simulink library "see_saw"  (R2013b)
settings: Solver=ode45  StartTime=0.0  StopTime=10.0  RelTol=1e-3
undefined symbols (not defined in the file): DiscIntNeverNeededParam, gcbh, K, R, realtime
libraries: legonxtlib x9
(part 2 of 2)

== stateflow chart see_saw/see_saw_mode_o ==
  state see_saw_mode
    entry:
    desired_tail = single(1.6);
    during:
    normalizedLight = processLight(sensors.light,lightCalib);
    PWM.tail = tail_controller(sensors.theta_T, desired_tail);
    DispTheta(states.phi);
    state light = processLight(rawLight,lightCalib) [function]
    state StandUp
      entry: debugFlag = uint16(602);
      initFlags.theta = single(1);
      initFlags.gyroReset = single(1);
      during:
      desired_tail = desired_tail + single(0.0008);
    state DispTheta(theta) [function]
    state cmd = phiController(phi,desiredPhi,battery) [function]
    state Balancing
      state SeesawLogic [parallel]
        settings: executionOrder=2
        state StationnaryBalance
          entry: debugFlag = uint16(603);
          desired_tail = single(0.5);
          initFlags.theta = single(0);
          initFlags.gyroReset = single(0);
          desired_states = balancerStates_Bus0;
        state Approach
          entry: debugFlag = uint16(604);
          during:
          turningPWM = lineTracker(single(-0.3), normalizedLight, single(1.3), sensors.battery);
          exit:
          turningPWM = single(0);
          state StartWalking
            entry:
            entry: debugFlag = uint16(605);
            des_vel = single(0.04);
            during:
            des_vel = des_vel+single(0.00024);
          state Walk
            entry: debugFlag = uint16(605);
          (default) -> StartWalking
          StartWalking -> Walk : [des_vel >= single(0.1)]
        state Seesaw
          state JumpOnIt
            entry:
            Speak;
            debugFlag = uint16(606);
            theta_ref = states.balancerStates.theta;
            phi_ref = states.phi;
            des_vel = single(0.15);
          state OnSeeSaw
            during:
            turningPWM = phiController(states.phi, phi_ref, sensors.battery);
            state GoingUP
              entry:
              entry: debugFlag = uint16(607);
              des_vel = single(0.1);
            state GoingBack
              entry:
              entry: debugFlag = uint16(608);
              des_vel = single(-0.1);
            state GoUpAgain
              entry:
              entry: debugFlag = uint16(609);
              des_vel = single(0.05);
              during:
              des_vel = des_vel + single(0.00024);
            state WaitForGettingDown
            GoingUP -> GoingBack : [states.balancerStates.theta >= theta_ref + single(9)]
            GoingBack -> GoUpAgain : [states.balancerStates.theta <= theta_ref + single(8.2)]
            GoUpAgain -> WaitForGettingDown : [des_vel >= 0.075]
          state Stop
            entry: debugFlag = uint16(610);
            des_vel = single(0.1);
            during:
            turningPWM = lineTracker(single(-0.3), normalizedLight, single(1.3), sensors.battery);
          state Warning
            entry: debugFlag = uint16(621);
            des_vel = single(0.1);
            during:
            turningPWM = lineTracker(single(-0.3), normalizedLight, single(1.3), sensors.battery);
          state DoneStates
            du: turningPWM = lineTracker(single(-0.3), normalizedLight, single(1.3), sensors.battery);
            state Done
              entry: debugFlag = uint16(611);
            state DecreaseSpeed
              en: des_vel = single(0.05);
              entry: debugFlag = uint16(612);
              du:
              des_vel = des_vel -single(0.0004);
            state ExitSeeSaw
              en:
              des_vel = single(0.025);
            Done -> DecreaseSpeed : [after(2,sec)]
            DecreaseSpeed -> ExitSeeSaw : [des_vel<single(0.025)]
          state Woops
            state Stabilize
              en:debugFlag = uint16(1120);
            state BackUpB1
              en: des_vel = single(-0.04);
              en:debugFlag = uint16(1121);
            state ReachedLine
              en:
              theta_l_0 = sensors.theta_L;
              debugFlag = uint16(1122);
              phi_ref = states.phi;
            state TurnNow
              en:
              des_vel = single(0);
              debugFlag = uint16(1123);
              des_turning = single(1.65);
              du:
              turningPWM = phiController(states.phi, (phi_ref - des_turning), sensors.battery);
            state GoOnYourMerryWay
              en:
              des_vel = single(0.02);
              %tracking = uint8(1);
              du:
              des_vel = des_vel+single(0.0004);
              turningPWM = lineTracker(single(-0.3), normalizedLight, single(1.3), sensors.battery);
              debugFlag = uint16(1124);
            (default) -> Stabilize : {FoundLine =uint8( 0);
                | %tracking = uint8(0);
                | %des_turning = single(0);
                | turningPWM = single(0);
                | des_vel = single(0);
                | }
            BackUpB1 -> ReachedLine : [normalizedLight >= single(0.5) ]
            Stabilize -> BackUpB1 : after(2,sec)
            ReachedLine -> TurnNow : [sensors.theta_L < theta_l_0-single(0.5)]
            TurnNow -> GoOnYourMerryWay : after(2.5,sec)
          (default) -> JumpOnIt
          JumpOnIt -> GoingUP : [states.balancerStates.theta >= theta_ref+single(1.57)]
          GoOnYourMerryWay -> ExitSeeSaw : [des_vel >=  single(0.025)]
          WaitForGettingDown -> Stop : [states.balancerStates.theta >= theta_ref + single(17)]
          Stop -> Warning [order 1] : [states.phi - phi_ref > single(0.5)]
          Warning -> Done [order 1] : [states.phi - phi_ref < single(-0.5)]
          Stop -> Done [order 2] : [states.phi - phi_ref < single(-0.5)]
          Warning -> Woops [order 2] : [states.phi - phi_ref > single(1.7)]
        state RaceDone
          entry: debugFlag = uint16(599);
          current_mode_status = OperationModeStatusEnum.SUCCESSFULLY_COMPLETED;
        (default) -> StationnaryBalance
        StationnaryBalance -> Approach : after(2,sec)
        Approach -> Seesaw : [states.balancerStates.theta_dot<single(-4)  && states.theta_dot_dot < single(-60) ]
        ExitSeeSaw -> RaceDone : after(0.5, sec)
      state After [parallel]
        during:
        forwardPWM = balance_ctrl(states.balancerStates, des_vel ,sensors.battery)
        PWM.left = forwardPWM - turningPWM;
        PWM.right = forwardPWM + turningPWM;
        settings: executionOrder=1
    state cmd = lineTracker(desiredLight,light,trackingPower,battery) [function]
    state Speak [function]
    state cmd = tail_controller(current,desired) [function]
    state cmd = balance_ctrl(balancerStates,desired_velocity,battery) [function]
    (default) -> StandUp
    StandUp -> Balancing : [desired_tail >=single(2.0) && sensors.theta_T >= single(2.0)]
  data: rawLight function_input single size=1; lightCalib function_input Bus: Light_Bus size=1; light function_output; theta function_input double size=1; cmd function_output; phi function_input single size=1; desiredPhi function_input single size=1; battery function_input double size=1; cmd function_output single size=1; desiredLight function_input single size=1; light function_input single size=1; trackingPower function_input single size=1; battery function_input double size=1; current function_input single size=1; desired function_input single size=1; cmd function_output single size=1; balancerStates function_input Bus: Balancer_States_Bus size=1; desired_velocity function_input single size=1; battery function_input double size=1; cmd function_output single size=1; states input Bus: States_Bus size=1; sensors input Bus: Sensors_Bus size=1; PWM output Bus: PWM_bus size=1; initFlags output Bus: Init_Bus size=1; debugFlag output uint16 size=1; desired_states local Bus: Balancer_States_Bus size=1; desired_tail local single size=1; current_mode_status data_store_memory; balancerStates_Bus0 parameter Bus: Balancer_States_Bus size=1; lightCalib data_store_memory; normalizedLight local single size=1; des_vel local single size=1; theta_ref local single size=1; forwardPWM local single size=1; turningPWM local single size=1; phi_ref local single; FoundLine local; des_turning local; theta_l_0 local

== stateflow chart see_saw/see_saw ==
  state see_saw_mode
    entry:
    desired_tail = single(1.6);
    desired_psi = single(0);
    theta_ref = single(0);
    during:
    normalizedLight = processLight(sensors.light,lightCalib);
    PWM.tail = tail_controller(sensors.theta_T, desired_tail);
    DispTheta(normalizedLight,turningPWM);
    state light = processLight(rawLight,lightCalib) [function]
    state StandUp
      entry: debugFlag = uint16(602);
      initFlags.theta = single(1);
      initFlags.gyroReset = single(1);
      during:
      desired_tail = desired_tail + single(0.0008);
    state DispTheta(light,turningPWM) [function]
    state cmd = phiController(phi,desiredPhi,battery) [function]
    state Balancing
      state SeesawLogic [parallel]
        settings: executionOrder=2
        state StationnaryBalance
          entry: debugFlag = uint16(603);
          desired_tail = single(0.5);
          initFlags.theta = single(0);
          initFlags.gyroReset = single(0);
          desired_states = balancerStates_Bus0;
        state Approach
          entry: debugFlag = uint16(604);
          during:
          turningPWM = lineTracker(single(-0.3), normalizedLight, single(1.3), sensors.battery);
          exit:
          turningPWM = single(0);
          state StartWalking
            entry:
            entry: debugFlag = uint16(605);
            des_vel = single(0.04);
            during:
            des_vel = des_vel+single(0.00024);
          state Walk
            entry: debugFlag = uint16(605);
          (default) -> StartWalking
          StartWalking -> Walk : [des_vel >= single(0.1)]
        state Seesaw
          state JumpOnIt
            entry:
            Speak;
            debugFlag = uint16(606);
            theta_ref = states.balancerStates.theta;
            phi_ref = states.phi;
            des_vel = single(0.15);
          state OnSeeSaw
            state GoingUP
              entry:
              debugFlag = uint16(607);des_vel = single(0.07);
              during:
              turningPWM = lineTracker(single(-0.6), normalizedLight, single(1), sensors.battery) + ...
              phiController(states.phi, phi_ref, sensors.battery);
            state GoingBack
              entry:
              debugFlag = uint16(608);
              des_vel = single(-0.1);
              during:
              turningPWM =phiController(states.phi, phi_ref, sensors.battery);
            state GoUpAgain
              entry:
              entry: debugFlag = uint16(609);
              des_vel = single(0.07);
              during:
              turningPWM = lineTracker(single(-0.6), normalizedLight, single(1), sensors.battery) + ...
              phiController(states.phi, phi_ref, sensors.battery);
              %des_vel = des_vel + single(0.00024);
            state WaitForGettingDown
              during:
              turningPWM = lineTracker(single(-0.6), normalizedLight, single(1), sensors.battery) + ...
              phiController(states.phi, phi_ref, sensors.battery);
            GoingUP -> GoingBack : [states.balancerStates.theta >= theta_ref + single(9.2)]
            GoingBack -> GoUpAgain : [states.balancerStates.theta <= theta_ref + single(8.2)]
          state Stop
            entry: debugFlag = uint16(610);
            des_vel = single(0.1);
            during:
            turningPWM = lineTracker(single(-0.3), normalizedLight, single(1.3), sensors.battery)+ ...
            phiController(states.phi, phi_ref, sensors.battery);
          state Warning
            entry: debugFlag = uint16(621);
            des_vel = single(0.05);
            during:
            turningPWM = lineTracker(single(-0.3), normalizedLight, single(1.6), sensors.battery);
          state DoneStates
            du: turningPWM = lineTracker(single(-0.3), normalizedLight, single(1.3), sensors.battery)+ ...
            phiController(states.phi, phi_ref, sensors.battery);
            state Done
              entry: debugFlag = uint16(611);
            state DecreaseSpeed
              en: des_vel = single(0.08);
              entry: debugFlag = uint16(612);
              du:
              des_vel = des_vel -single(0.0004);
            state ExitSeeSaw
              en:
              des_vel = single(0.08)
            Done -> DecreaseSpeed : [after(2,sec)]
            DecreaseSpeed -> ExitSeeSaw : %[des_vel<single(0.08)]
          state Woops
            state Stabilize
              en:debugFlag = uint16(1120);
            state BackUpB1
              en: des_vel = single(-0.05);
              en:debugFlag = uint16(1121);
            state ReachedLine
              en:
              theta_l_0 = sensors.theta_L;
              debugFlag = uint16(1122);
              phi_ref = states.phi;
            state TurnNow
              en:
              des_vel = single(0);
              debugFlag = uint16(1123);
              des_turning = single(1.65);
              du:
              turningPWM = phiController(states.phi, (phi_ref - des_turning), sensors.battery);
            state GoOnYourMerryWay
              en:
              des_vel = single(0.02);
              turningPWM = lineTracker(single(-0.3), normalizedLight, single(1.3), sensors.battery);
              du:
              des_vel = des_vel+single(0.0004);
              turningPWM = lineTracker(single(-0.3), normalizedLight, single(1.3), sensors.battery);
              debugFlag = uint16(1124);
            (default) -> Stabilize : {FoundLine =uint8( 0);
                | %tracking = uint8(0);
                | %des_turning = single(0);
                | turningPWM = single(0);
                | des_vel = single(0);
                | }
            BackUpB1 -> ReachedLine : [normalizedLight >= single(0.5) ]
            Stabilize -> BackUpB1 : after(2,sec)
            ReachedLine -> TurnNow : [sensors.theta_L < theta_l_0-single(0.5)]
            TurnNow -> GoOnYourMerryWay : after(2.5,sec)
          (default) -> JumpOnIt
          JumpOnIt -> GoingUP : [states.balancerStates.theta >= theta_ref+single(1.57)]
          GoUpAgain -> Stop : [states.balancerStates.theta >= theta_ref + single(17)]
          GoOnYourMerryWay -> ExitSeeSaw : [des_vel >=  single(0.04)]
          Stop -> Warning [order 1] : [states.phi - phi_ref > single(0.5)]
          Warning -> Done [order 1] : [states.phi - phi_ref < single(-0.2)]
          Stop -> Done [order 2] : [states.phi - phi_ref < single(0)]
          Warning -> Woops [order 2] : [states.phi - phi_ref > single(1.7)]
        state Parking
          en,du:
          turningPWM = single(2)*lineTracker(single(-0.3), normalizedLight, single(1), sensors.battery) + phiController(states.phi, phi_ref, sensors.battery);
          state DropTailAndGrey
            state TailDrop
              entry: debugFlag = uint16(801);
              during:
              desired_tail = desired_tail + single(0.1);
            state LookForGrey
              entry: debugFlag = uint16(803);
            (default) -> TailDrop
            TailDrop -> LookForGrey : [desired_tail > single(1.6)]
          state WaitAndCount
            entry: debugFlag = uint16(804);
          state FallBack
            entry: debugFlag = uint16(805);
            desired_psi = single(-0.15);
          state DoneWithParking
            entry: debugFlag = uint16(806);
            exit:
            PWM.left = single(0);
            PWM.right = single(0);
          (default) -> DropTailAndGrey
          LookForGrey -> FallBack : [states.balancerStates.theta >= theta_ref + single(32)]
          WaitAndCount -> WaitAndCount [order 1] : [-100*normalizedLight <= single(-12)]
          WaitAndCount -> FallBack [order 2] : after(0.3,sec)
          FallBack -> DoneWithParking : after(0.2,sec)
        state RaceDone
          entry: debugFlag = uint16(599);
          current_mode_status = OperationModeStatusEnum.SUCCESSFULLY_COMPLETED;
        (default) -> StationnaryBalance
        StationnaryBalance -> Approach : after(2,sec)
        Approach -> Seesaw : [states.balancerStates.theta_dot<single(-4)  && states.theta_dot_dot < single(-60) ]
        ExitSeeSaw -> Parking : after(0.1,sec)
      state After [parallel]
        during:
        forwardPWM = balance_ctrl(states.balancerStates, des_vel ,sensors.battery, desired_psi)
        if (debugFlag~= uint16(806))
        PWM.left = forwardPWM - turningPWM;
        PWM.right = forwardPWM + turningPWM;
        else
        PWM.left = single(0);
        PWM.right = single(0);
        end
        settings: executionOrder=1
    state cmd = lineTracker(desiredLight,light,trackingPower,battery) [function]
    state Speak [function]
    state cmd = tail_controller(current,desired) [function]
    state cmd = balance_ctrl(balancerStates,desired_velocity,battery,desired_psi) [function]
    (default) -> StandUp
    StandUp -> Balancing : [desired_tail >=single(2.0) && sensors.theta_T >= single(2.0)]
  data: rawLight function_input single size=1; lightCalib function_input Bus: Light_Bus size=1; light function_output; light function_input double size=1; turningPWM function_input double size=1; cmd function_output; phi function_input single size=1; desiredPhi function_input single size=1; battery function_input double size=1; cmd function_output single size=1; desiredLight function_input single size=1; light function_input single size=1; trackingPower function_input single size=1; battery function_input double size=1; current function_input single size=1; desired function_input single size=1; cmd function_output single size=1; balancerStates function_input Bus: Balancer_States_Bus size=1; desired_velocity function_input single size=1; battery function_input double size=1; cmd function_output single size=1; desired_psi function_input single size=1; states input Bus: States_Bus size=1; sensors input Bus: Sensors_Bus size=1; PWM output Bus: PWM_bus size=1; initFlags output Bus: Init_Bus size=1; debugFlag output uint16 size=1; desired_states local Bus: Balancer_States_Bus size=1; desired_tail local single size=1; current_mode_status data_store_memory; balancerStates_Bus0 parameter Bus: Balancer_States_Bus size=1; lightCalib data_store_memory; normalizedLight local single size=1; des_vel local single size=1; theta_ref local single size=1; forwardPWM local single size=1; turningPWM local single size=1; phi_ref local single; FoundLine local; des_turning local; theta_l_0 local; desired_psi local

== stateflow chart see_saw/see_saw_8262013 ==
  state see_saw_mode
    entry:
    desired_tail = single(1.6);
    desired_psi = single(0);
    theta_ref = single(0);
    during:
    normalizedLight = processLight(sensors.light,lightCalib);
    PWM.tail = tail_controller(sensors.theta_T, desired_tail);
    DispTheta(states.balancerStates.theta - theta_ref);
    state light = processLight(rawLight,lightCalib) [function]
    state StandUp
      entry: debugFlag = uint16(602);
      initFlags.theta = single(1);
      initFlags.gyroReset = single(1);
      during:
      desired_tail = desired_tail + single(0.0008);
    state DispTheta(theta) [function]
    state cmd = phiController(phi,desiredPhi,battery) [function]
    state Balancing
      state SeesawLogic [parallel]
        settings: executionOrder=2
        state StationnaryBalance
          entry: debugFlag = uint16(603);
          desired_tail = single(0.5);
          initFlags.theta = single(0);
          initFlags.gyroReset = single(0);
          desired_states = balancerStates_Bus0;
        state Approach
          entry: debugFlag = uint16(604);
          during:
          turningPWM = lineTracker(single(-0.3), normalizedLight, single(1.3), sensors.battery);
          exit:
          turningPWM = single(0);
          state StartWalking
            entry:
            entry: debugFlag = uint16(605);
            des_vel = single(0.04);
            during:
            des_vel = des_vel+single(0.00024);
          state Walk
            entry: debugFlag = uint16(605);
          (default) -> StartWalking
          StartWalking -> Walk : [des_vel >= single(0.1)]
        state Seesaw
          state JumpOnIt
            entry:
            Speak;
            debugFlag = uint16(606);
            theta_ref = states.balancerStates.theta;
            phi_ref = states.phi;
            des_vel = single(0.15);
          state OnSeeSaw
            during:
            turningPWM = phiController(states.phi, phi_ref, sensors.battery);
            state GoingUP
              entry:
              entry: debugFlag = uint16(607);
              des_vel = single(0.1);
            state GoingBack
              entry:
              entry: debugFlag = uint16(608);
              des_vel = single(-0.1);
            state GoUpAgain
              entry:
              entry: debugFlag = uint16(609);
              des_vel = single(0.05);
              during:
              des_vel = des_vel + single(0.00024);
            state WaitForGettingDown
            GoingUP -> GoingBack : [states.balancerStates.theta >= theta_ref + single(9)]
            GoingBack -> GoUpAgain : [states.balancerStates.theta <= theta_ref + single(8.2)]
            GoUpAgain -> WaitForGettingDown : [des_vel >= 0.075]
          state Stop
            entry: debugFlag = uint16(610);
            des_vel = single(0.1);
            during:
            turningPWM = lineTracker(single(-0.3), normalizedLight, single(1.3), sensors.battery);
          state Warning
            entry: debugFlag = uint16(621);
            des_vel = single(0.05);
            during:
            turningPWM = lineTracker(single(-0.3), normalizedLight, single(1.6), sensors.battery);
          state DoneStates
            du: turningPWM = lineTracker(single(-0.3), normalizedLight, single(1.3), sensors.battery);
            state Done
              entry: debugFlag = uint16(611);
            state DecreaseSpeed
              en: des_vel = single(0.08);
              entry: debugFlag = uint16(612);
              du:
              des_vel = des_vel -single(0.0004);
            state ExitSeeSaw
              en:
              des_vel = single(0.08)
            Done -> DecreaseSpeed : [after(2,sec)]
            DecreaseSpeed -> ExitSeeSaw : %[des_vel<single(0.08)]
          state Woops
            state Stabilize
              en:debugFlag = uint16(1120);
            state BackUpB1
              en: des_vel = single(-0.05);
              en:debugFlag = uint16(1121);
            state ReachedLine
              en:
              theta_l_0 = sensors.theta_L;
              debugFlag = uint16(1122);
              phi_ref = states.phi;
            state TurnNow
              en:
              des_vel = single(0);
              debugFlag = uint16(1123);
              des_turning = single(1.65);
              du:
              turningPWM = phiController(states.phi, (phi_ref - des_turning), sensors.battery);
            state GoOnYourMerryWay
              en:
              des_vel = single(0.02);
              turningPWM = lineTracker(single(-0.3), normalizedLight, single(1.3), sensors.battery);
              du:
              des_vel = des_vel+single(0.0004);
              turningPWM = lineTracker(single(-0.3), normalizedLight, single(1.3), sensors.battery);
              debugFlag = uint16(1124);
            (default) -> Stabilize : {FoundLine =uint8( 0);
                | %tracking = uint8(0);
                | %des_turning = single(0);
                | turningPWM = single(0);
                | des_vel = single(0);
                | }
            BackUpB1 -> ReachedLine : [normalizedLight >= single(0.5) ]
            Stabilize -> BackUpB1 : after(2,sec)
            ReachedLine -> TurnNow : [sensors.theta_L < theta_l_0-single(0.5)]
            TurnNow -> GoOnYourMerryWay : after(2.5,sec)
          (default) -> JumpOnIt
          JumpOnIt -> GoingUP : [states.balancerStates.theta >= theta_ref+single(1.57)]
          GoOnYourMerryWay -> ExitSeeSaw : [des_vel >=  single(0.04)]
          WaitForGettingDown -> Stop : [states.balancerStates.theta >= theta_ref + single(17)]
          Stop -> Warning [order 1] : [states.phi - phi_ref > single(0.5)]
          Warning -> Done [order 1] : [states.phi - phi_ref < single(-0.2)]
          Stop -> Done [order 2] : [states.phi - phi_ref < single(-0.2)]
          Warning -> Woops [order 2] : [states.phi - phi_ref > single(1.7)]
        state Parking
          en,du:
          turningPWM = single(2)*lineTracker(single(-0.3), normalizedLight, single(1), sensors.battery) + phiController(states.phi, phi_ref, sensors.battery);
          state DropTailAndGrey
            state TailDrop
              entry: debugFlag = uint16(801);
              during:
              desired_tail = desired_tail + single(0.1);
            state LookForGrey
              entry: debugFlag = uint16(803);
            (default) -> TailDrop
            TailDrop -> LookForGrey : [desired_tail > single(1.6)]
          state WaitAndCount
            entry: debugFlag = uint16(804);
          state FallBack
            entry: debugFlag = uint16(805);
            desired_psi = single(-0.15);
          state DoneWithParking
            entry: debugFlag = uint16(806);
            exit:
            PWM.left = single(0);
            PWM.right = single(0);
          (default) -> DropTailAndGrey
          LookForGrey -> FallBack : [states.balancerStates.theta >= theta_ref + single(33)]
          WaitAndCount -> WaitAndCount [order 1] : [-100*normalizedLight <= single(-12)]
          WaitAndCount -> FallBack [order 2] : after(0.3,sec)
          FallBack -> DoneWithParking : after(0.2,sec)
        state RaceDone
          entry: debugFlag = uint16(599);
          current_mode_status = OperationModeStatusEnum.SUCCESSFULLY_COMPLETED;
        (default) -> StationnaryBalance
        StationnaryBalance -> Approach : after(2,sec)
        Approach -> Seesaw : [states.balancerStates.theta_dot<single(-4)  && states.theta_dot_dot < single(-60) ]
        ExitSeeSaw -> Parking : after(0.1,sec)
      state After [parallel]
        during:
        forwardPWM = balance_ctrl(states.balancerStates, des_vel ,sensors.battery, desired_psi)
        if (debugFlag~= uint16(806))
        PWM.left = forwardPWM - turningPWM;
        PWM.right = forwardPWM + turningPWM;
        else
        PWM.left = single(0);
        PWM.right = single(0);
        end
        settings: executionOrder=1
    state cmd = lineTracker(desiredLight,light,trackingPower,battery) [function]
    state Speak [function]
    state cmd = tail_controller(current,desired) [function]
    state cmd = balance_ctrl(balancerStates,desired_velocity,battery,desired_psi) [function]
    (default) -> StandUp
    StandUp -> Balancing : [desired_tail >=single(2.0) && sensors.theta_T >= single(2.0)]
  data: rawLight function_input single size=1; lightCalib function_input Bus: Light_Bus size=1; light function_output; theta function_input double size=1; cmd function_output; phi function_input single size=1; desiredPhi function_input single size=1; battery function_input double size=1; cmd function_output single size=1; desiredLight function_input single size=1; light function_input single size=1; trackingPower function_input single size=1; battery function_input double size=1; current function_input single size=1; desired function_input single size=1; cmd function_output single size=1; balancerStates function_input Bus: Balancer_States_Bus size=1; desired_velocity function_input single size=1; battery function_input double size=1; cmd function_output single size=1; desired_psi function_input single size=1; states input Bus: States_Bus size=1; sensors input Bus: Sensors_Bus size=1; PWM output Bus: PWM_bus size=1; initFlags output Bus: Init_Bus size=1; debugFlag output uint16 size=1; desired_states local Bus: Balancer_States_Bus size=1; desired_tail local single size=1; current_mode_status data_store_memory; balancerStates_Bus0 parameter Bus: Balancer_States_Bus size=1; lightCalib data_store_memory; normalizedLight local single size=1; des_vel local single size=1; theta_ref local single size=1; forwardPWM local single size=1; turningPWM local single size=1; phi_ref local single; FoundLine local; des_turning local; theta_l_0 local; desired_psi local

== stateflow chart see_saw/see_saw_atomic ==
  state see_saw_mode
    entry:
    desired_tail = single(0);
    desired_psi = single(0);
    theta_ref = single(0);
    during:
    normalizedLight = processLight(sensors.light,lightCalib);
    PWM.tail = tail_controller(sensors.theta_T, desired_tail);
    DispTheta(normalizedLight,turningPWM);
    state StandUp
      entry:
      debugFlag = uint16(602);
      initFlags.theta = single(1);
      initFlags.gyroReset = single(1);
    state Balancing
      state SeesawLogic [parallel]
        settings: executionOrder=1
        state StationnaryBalance
          entry:
          Speak;
          debugFlag = uint16(603);
          initFlags.theta = single(0);
          initFlags.gyroReset = single(0);
          desired_states = balancerStates_Bus0;
        state Approach
          entry: debugFlag = uint16(604);
          turningPWM = single(0);
          trackingPower = single(0);
          bias = single(0.3);
          Speak;
          during:
          turningPWM = lineTracker(bias, normalizedLight, trackingPower, sensors.battery);
          exit:
          turningPWM = single(0);
          state manageBias [parallel]
            settings: executionOrder=3
            state Start
              during:
              bias = bias - single(0.6/500);
            state done
              entry: bias = single(-0.3);
            (default) -> see_saw_mode.Balancing.SeesawLogic.Approach.manageBias.Start
            see_saw_mode.Balancing.SeesawLogic.Approach.manageBias.Start -> done : [bias <= single(-0.3)]
          state Turning [parallel]
            settings: executionOrder=1
            state Start
              during:
              trackingPower = trackingPower+single(1.3/250);
            state fullTrack
              entry: trackingPower = single(1.3);
            (default) -> see_saw_mode.Balancing.SeesawLogic.Approach.Turning.Start
            see_saw_mode.Balancing.SeesawLogic.Approach.Turning.Start -> fullTrack : [trackingPower >= single(1.3)]
          state Forward [parallel]
            settings: executionOrder=2
            state StartWalking
              entry: debugFlag = uint16(605);
              des_vel = single(0);
              during:
              des_vel = des_vel+single(0.00024);
            state Walk
              entry: debugFlag = uint16(605);
            (default) -> StartWalking
            StartWalking -> Walk : [des_vel >= single(0.1)]
        state Seesaw
          state JumpOnIt
            entry:
            Speak;
            debugFlag = uint16(606);
            theta_ref = states.balancerStates.theta;
            phi_ref = states.phi;
            des_vel = single(0.15);
          state OnSeeSaw
            state GoingUP
              entry:
              debugFlag = uint16(607);des_vel = single(0.07);
              during:
              turningPWM = lineTracker(single(-0.6), normalizedLight, single(1), sensors.battery) + ...
              phiController(states.phi, phi_ref, sensors.battery);
            state GoingBack
              entry:
              debugFlag = uint16(608);
              des_vel = single(-0.1);
              during:
              turningPWM =phiController(states.phi, phi_ref, sensors.battery);
            state GoUpAgain
              entry:
              entry: debugFlag = uint16(609);
              des_vel = single(0.07);
              during:
              turningPWM = lineTracker(single(-0.6), normalizedLight, single(1), sensors.battery) + ...
              phiController(states.phi, phi_ref, sensors.battery);
              %des_vel = des_vel + single(0.00024);
            state WaitForGettingDown
              during:
              turningPWM = lineTracker(single(-0.6), normalizedLight, single(1), sensors.battery) + ...
              phiController(states.phi, phi_ref, sensors.battery);
            GoingUP -> GoingBack : [states.balancerStates.theta >= theta_ref + single(9.2)]
            GoingBack -> GoUpAgain : [states.balancerStates.theta <= theta_ref + single(8.2)]
          state Stop
            entry: debugFlag = uint16(610);
            des_vel = single(0.1);
            during:
            turningPWM = lineTracker(single(-0.3), normalizedLight, single(1.3), sensors.battery)+ ...
            phiController(states.phi, phi_ref, sensors.battery);
          state Warning
            entry: debugFlag = uint16(621);
            des_vel = single(0.05);
            during:
            turningPWM = lineTracker(single(-0.3), normalizedLight, single(1.6), sensors.battery);
          state DoneStates
            du: turningPWM = lineTracker(single(-0.1), normalizedLight, single(1.3), sensors.battery)+ ...
            phiController(states.phi, phi_ref, sensors.battery);
            state Done
              entry: debugFlag = uint16(611);
            state DecreaseSpeed
              en: des_vel = single(0.08);
              entry: debugFlag = uint16(612);
              du:
              des_vel = des_vel -single(0.0004);
            state ExitSeeSaw
              en:
              des_vel = single(0.08)
            Done -> DecreaseSpeed : [after(2,sec)]
            DecreaseSpeed -> ExitSeeSaw : %[des_vel<single(0.08)]
          state Woops
            state Stabilize
              en:debugFlag = uint16(1120);
            state BackUpB1
              en: des_vel = single(-0.05);
              en:debugFlag = uint16(1121);
            state ReachedLine
              en:
              theta_l_0 = sensors.theta_L;
              debugFlag = uint16(1122);
              phi_ref = states.phi;
            state TurnNow
              en:
              des_vel = single(0);
              debugFlag = uint16(1123);
              des_turning = single(1.65);
              du:
              turningPWM = phiController(states.phi, (phi_ref - des_turning), sensors.battery);
            state GoOnYourMerryWay
              en:
              des_vel = single(0.02);
              turningPWM = lineTracker(single(-0.3), normalizedLight, single(1.3), sensors.battery);
              du:
              des_vel = des_vel+single(0.0004);
              turningPWM = lineTracker(single(-0.3), normalizedLight, single(1.3), sensors.battery);
              debugFlag = uint16(1124);
            (default) -> Stabilize : {FoundLine =uint8( 0);
                | %tracking = uint8(0);
                | %des_turning = single(0);
                | turningPWM = single(0);
                | des_vel = single(0);
                | }
            BackUpB1 -> ReachedLine : [normalizedLight >= single(0.5) ]
            Stabilize -> BackUpB1 : after(2,sec)
            ReachedLine -> TurnNow : [sensors.theta_L < theta_l_0-single(0.5)]
            TurnNow -> GoOnYourMerryWay : after(2.5,sec)
          (default) -> JumpOnIt
          JumpOnIt -> GoingUP : [states.balancerStates.theta >= theta_ref+single(1.57)]
          GoUpAgain -> Stop : [states.balancerStates.theta >= theta_ref + single(17)]
          GoOnYourMerryWay -> ExitSeeSaw : [des_vel >=  single(0.04)]
          Stop -> Warning [order 1] : [states.phi - phi_ref > single(0.5)]
          Warning -> Done [order 1] : [states.phi - phi_ref < single(-0.2)]
          Stop -> Done [order 2] : [states.phi - phi_ref < single(0)]
          Warning -> Woops [order 2] : [states.phi - phi_ref > single(1.7)]
        state Parking
          en,du:
          turningPWM = single(2)*lineTracker(single(-0.1), normalizedLight, single(1), sensors.battery) + phiController(states.phi, phi_ref, sensors.battery);
          state DropTailAndGrey
            state TailDrop
              entry: debugFlag = uint16(801);
              during:
              desired_tail = desired_tail + single(0.1);
            state LookForGrey
              entry: debugFlag = uint16(803);
            (default) -> TailDrop
            TailDrop -> LookForGrey : [desired_tail > single(1.6)]
          state WaitAndCount
            entry: debugFlag = uint16(804);
          state FallBack
            entry: debugFlag = uint16(805);
            desired_psi = single(-0.15);
          state DoneWithParking
            entry: debugFlag = uint16(806);
            exit:
            PWM.left = single(0);
            PWM.right = single(0);
          (default) -> DropTailAndGrey
          LookForGrey -> FallBack : [states.balancerStates.theta >= theta_ref + single(32)]
          WaitAndCount -> WaitAndCount [order 1] : [-100*normalizedLight <= single(-12)]
          WaitAndCount -> FallBack [order 2] : after(0.3,sec)
          FallBack -> DoneWithParking : after(0.2,sec)
        state RaceDone
          entry: debugFlag = uint16(599);
          current_mode_status = OperationModeStatusEnum.SUCCESSFULLY_COMPLETED;
        (default) -> StationnaryBalance
        StationnaryBalance -> Approach : after(1,sec)
        Approach -> Seesaw : [states.balancerStates.theta_dot<single(-4)  && states.theta_dot_dot < single(-60) ]
        ExitSeeSaw -> Parking : after(0.1,sec)
      state After [parallel]
        during:
        forwardPWM = balance_ctrl(states.balancerStates, des_vel ,sensors.battery, desired_psi)
        if (debugFlag~= uint16(806))
        PWM.left = forwardPWM - turningPWM;
        PWM.right = forwardPWM + turningPWM;
        else
        PWM.left = single(0);
        PWM.right = single(0);
        end
        settings: executionOrder=2
    state light = processLight(rawLight,lightCalib) [function]
    state DispTheta(light,turningPWM) [function]
    state cmd = phiController(phi,desiredPhi,battery) [function]
    state cmd = lineTracker(desiredLight,light,trackingPower,battery) [function]
    state Speak [function]
    state cmd = tail_controller(current,desired) [function]
    state cmd = balance_ctrl(balancerStates,desired_velocity,battery,desired_psi) [function]
    (default) -> StandUp
    StandUp -> Balancing
  data: rawLight function_input single size=1; lightCalib function_input Bus: Light_Bus size=1; light function_output; light function_input double size=1; turningPWM function_input double size=1; cmd function_output; phi function_input single size=1; desiredPhi function_input single size=1; battery function_input double size=1; cmd function_output single size=1; desiredLight function_input single size=1; light function_input single size=1; trackingPower function_input single size=1; battery function_input double size=1; current function_input single size=1; desired function_input single size=1; cmd function_output single size=1; balancerStates function_input Bus: Balancer_States_Bus size=1; desired_velocity function_input single size=1; battery function_input double size=1; cmd function_output single size=1; desired_psi function_input single size=1; states input Bus: States_Bus size=1; sensors input Bus: Sensors_Bus size=1; PWM output Bus: PWM_bus size=1; initFlags output Bus: Init_Bus size=1; debugFlag output uint16 size=1; desired_states local Bus: Balancer_States_Bus size=1; desired_tail local single size=1; current_mode_status data_store_memory; balancerStates_Bus0 parameter Bus: Balancer_States_Bus size=1; lightCalib data_store_memory; normalizedLight local single size=1; des_vel local single size=1; theta_ref local single size=1; forwardPWM local single size=1; turningPWM local single size=1; phi_ref local single; FoundLine local; des_turning local; theta_l_0 local; desired_psi local; trackingPower local; bias local
